simulink model "KVHSerial02"  (R2013a)
settings: Solver=FixedStepDiscrete  StartTime=0.0  StopTime=inf  FixedStep=0.001  RelTol=1e-3
undefined symbols (not defined in the file or in its folder): standard, XOFF, XON
libraries: simulink x2, xpcseriallib x1, xpclib x1, speedgoatlib x1
settings Model: BufferReuse=off  Creator=bgbuss  LastModifiedBy=bgbuss
settings DataIOCC: LimitDataPoints=off  SignalLoggingSaveFormat=ModelDataLogs
settings OptimizationCC: BlockReduction=off  OptimizeBlockIOStorage=off  BufferReuse=off  ExpressionFolding=off  ExpressionDepthLimit=2147483647  LocalBlockOutputs=off
settings DebuggingCC: UnderspecifiedInitializationDetection=Simplified  FcnCallInpInsideContextMsg=EnableAllAsWarning  StrictBusMsg=ErrorOnBusTreatedAsVector
settings HardwareCC: ProdIntDivRoundTo=Zero  ProdEndianess=LittleEndian  ProdHWDeviceType=Generic->32-bit x86 compatible
settings RTWCC: SystemTargetFile=xpctarget.tlc  TemplateMakefile=xpc_default_tmf  Description=xPC Target  ProcessScript=xpctarget_make_rtw_hook
settings xpcTargetCC: TargetFcnLib=ansi_tfl_table_tmw.mat  CodeReplacementLibrary=XPC_BLAS  ParMdlRefBuildCompliant=on  ConcurrentExecutionCompliant=on  CombineSignalStateStructs=off  MATLABClassNameForMDSCustomization=xpcAperiodicCustomization  GRTInterface=on  GenerateAllocFcn=off  RL32LogBufSizeModifier=10000000  xPCTaskExecutionProfile=off  xPCRL32EventNumber=5000  xPCisModelTimeout=off  xPCModelTimeoutSecs=10  xPCLoadParamSetFile=off  xPCConcurrentTasks=off  xPCEnableSFAnimation=off

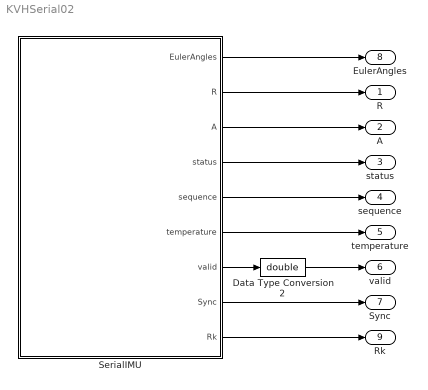
== system KVHSerial02 ==
  Data Type Conversion2 : DataTypeConversion  OutDataTypeStr=double
  SerialIMU : Subsystem
  R : Outport
  A : Outport  Port=2
  status : Outport  Port=3
  sequence : Outport  Port=4
  temperature : Outport  Port=5
  valid : Outport  Port=6
  Sync : Outport  Port=7
  EulerAngles : Outport  Port=8
  Rk : Outport  Port=9
  wires:
  SerialIMU/7(valid) -> Data Type Conversion2/1
  SerialIMU/3(A) -> A/1
  SerialIMU/2(R) -> R/1
  SerialIMU/4(status) -> status/1
  SerialIMU/5(sequence) -> sequence/1
  SerialIMU/6(temperature) -> temperature/1
  SerialIMU/8(Sync) -> Sync/1
  SerialIMU/1(EulerAngles) -> EulerAngles/1
  SerialIMU/9(Rk) -> Rk/1
  Data Type Conversion2/1 -> valid/1

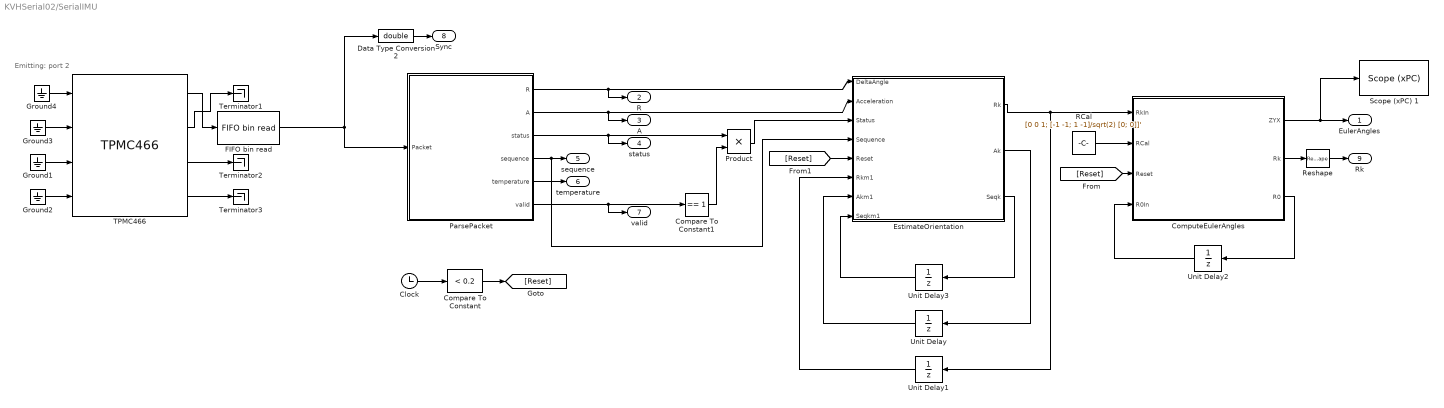
== system KVHSerial02/SerialIMU ==
  note: Emitting: port 2
  Clock : Clock
  Compare To Constant : simulink/Logic and Bit Operations/Compare To Constant  relop=<  const=0.2  OutDataTypeStr=uint8
  Compare To Constant1 : simulink/Logic and Bit Operations/Compare To Constant  relop===  const=1  OutDataTypeStr=uint8
  ComputeEulerAngles : MATLAB Function  TreatAsAtomicUnit=on
  Data Type Conversion2 : DataTypeConversion  OutDataTypeStr=double
  EstimateOrientation : MATLAB Function  TreatAsAtomicUnit=on
  "FIFO bin read " : xpcseriallib/FIFO bin read   header={char([254 129 255 85])}  lengths=[36]  hold=Zero output if no new data  enable=off  maxsize=64  outputtype=8 bit uint null terminated  sampletime=0.001
  Ground{1..4} (4 alike) : Ground
  ParsePacket : Subsystem
  Product : Product  RndMeth=Zero
  RCal : Constant  Value=[0 0 1; [-1 -1; 1 -1]/sqrt(2) [0; 0]]'
  Reshape : Reshape
  Scope (xPC) 1 : xpclib/Misc./Scope (xPC)   scopeno=1  scopetype=Target  autostart=on  viewmode=Graphical rolling  formatstr='%15.6f'  grid=on  ylimits=[-pi pi]  nosamples=500  noprepostsamples=0  interleave=10  triggermode=FreeRun  triggersignal=1  trigsignalfromport=off  triggerlevel=0.0  triggerslope=Either  triggerscope=1  triggersample=0  filename=data.dat  mode=Lazy  writesize=512  autorestart=off  dynamicfilemode=off  maxwritefilesize=512*1024^2
  TPMC466 : speedgoatlib/IO503/TPMC466  group=Basic Setup  port=1  irqnum=9  slot=-1  transceiver1=RS422  standard1=on  baud1=921600  bauddivisor1=1  sampling1=16x (standard)  prescale1=off  parity1=None  ndata1=8  nstop1=1  rlevel1=1  hwmode1=none  swmode1=none  xonchar1=17  xoffchar1=19  rs485auto1=off  rs485delay1=1  xmtfifosize1=1024  xmtdatatype1=8 bit uint null terminated  rcvfifosize1=1024  transceiver2=RS485 half-duplex  standard2=on  baud2=2764800  bauddivisor2=1  sampling2=16x (standard)  prescale2=off  parity2=None  ndata2=8  nstop2=1  rlevel2=quarter full (16)  hwmode2=none  swmode2=XON/XOFF  xonchar2=17  xoffchar2=19  rs485auto2=on  rs485delay2=1  xmtfifosize2=1024  xmtdatatype2=8 bit uint null terminated  rcvfifosize2=1024  transceiver3=RS485 half-duplex  standard3=on  baud3=115200  bauddivisor3=1  sampling3=16x (standard)  prescale3=off  parity3=None  ndata3=8  nstop3=1  rlevel3=half full (32)  hwmode3=none  swmode3=none  xonchar3=17  xoffchar3=19  rs485auto3=off  rs485delay3=0  xmtfifosize3=1024  xmtdatatype3=8 bit uint null terminated  rcvfifosize3=1024  transceiver4=RS485 half-duplex  standard4=on  baud4=115200  bauddivisor4=1  sampling4=16x (standard)  prescale4=off  parity4=None  ndata4=8  nstop4=1  rlevel4=half full (32)  hwmode4=none  swmode4=none  xonchar4=17  xoffchar4=19  rs485auto4=off  rs485delay4=0  xmtfifosize4=1024  xmtdatatype4=8 bit uint null terminated  rcvfifosize4=1024
  Terminator1 : Terminator
  Terminator2 : Terminator
  Terminator3 : Terminator
  Unit Delay : UnitDelay  InitialCondition=[0; 0; 0]  SampleTime=-1
  Unit Delay1 : UnitDelay  InitialCondition=zeros(3,3)  SampleTime=-1
  Unit Delay2 : UnitDelay  InitialCondition=zeros(3,3)  SampleTime=-1
  Unit Delay3 : UnitDelay  SampleTime=-1
  EulerAngles : Outport
  R : Outport  Port=2
  A : Outport  Port=3
  status : Outport  Port=4
  sequence : Outport  Port=5
  temperature : Outport  Port=6
  valid : Outport  Port=7
  Sync : Outport  Port=8
  Rk : Outport  Port=9
  wires:
  ParsePacket/2(A) -> EstimateOrientation/2(Acceleration), A/1
  ParsePacket/1(R) -> EstimateOrientation/1(DeltaAngle), R/1
  ParsePacket/3(status) -> status/1, Product/1
  ParsePacket/4(sequence) -> EstimateOrientation/4(Sequence), sequence/1
  ParsePacket/5(temperature) -> temperature/1
  "FIFO bin read "/1 -> ParsePacket/1(Packet), Data Type Conversion2/1
  ParsePacket/6(valid) -> valid/1, Compare To Constant1/1
  Data Type Conversion2/1 -> Sync/1
  EstimateOrientation/2(Ak) -> Unit Delay/1
  Unit Delay/1 -> EstimateOrientation/7(Akm1)
  EstimateOrientation/1(Rk) -> Unit Delay1/1, ComputeEulerAngles/1(RkIn)
  Unit Delay1/1 -> EstimateOrientation/6(Rkm1)
  [Reset] -> EstimateOrientation/5(Reset)
  RCal/1 -> ComputeEulerAngles/2(RCal)
  Unit Delay2/1 -> ComputeEulerAngles/4(R0In)
  ComputeEulerAngles/1(ZYX) -> Scope (xPC) 1/1, EulerAngles/1
  ComputeEulerAngles/3(R0) -> Unit Delay2/1
  ComputeEulerAngles/2(Rk) -> Reshape/1
  [Reset] -> ComputeEulerAngles/3(Reset)
  Clock/1 -> Compare To Constant/1
  Compare To Constant/1 -> [Reset]
  Reshape/1 -> Rk/1
  Product/1 -> EstimateOrientation/3(Status)
  Compare To Constant1/1 -> Product/2
  Ground4/1 -> TPMC466/1
  Ground3/1 -> TPMC466/2
  Ground1/1 -> TPMC466/3
  Ground2/1 -> TPMC466/4
  TPMC466/3 -> Terminator2/1
  TPMC466/4 -> Terminator3/1
  TPMC466/1 -> "FIFO bin read "/1
  TPMC466/2 -> Terminator1/1
  EstimateOrientation/3(Seqk) -> Unit Delay3/1
  Unit Delay3/1 -> EstimateOrientation/8(Seqkm1)

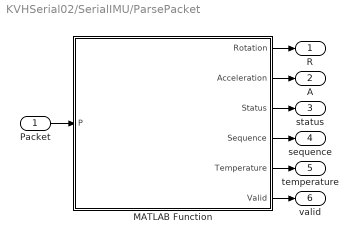
== system KVHSerial02/SerialIMU/ParsePacket ==
  Packet : Inport
  MATLAB Function : MATLAB Function  TreatAsAtomicUnit=on
  R : Outport
  A : Outport  Port=2
  status : Outport  Port=3
  sequence : Outport  Port=4
  temperature : Outport  Port=5
  valid : Outport  Port=6
  wires:
  MATLAB Function/1(Rotation) -> R/1
  MATLAB Function/2(Acceleration) -> A/1
  MATLAB Function/3(Status) -> status/1
  Packet/1 -> MATLAB Function/1(P)
  MATLAB Function/4(Sequence) -> sequence/1
  MATLAB Function/5(Temperature) -> temperature/1
  MATLAB Function/6(Valid) -> valid/1

== matlab function KVHSerial02/SerialIMU/ComputeEulerAngles ==
  data: RkIn input; RCal input; Reset input; R0In input; ZYX output; Rk output; R0 output
function [ZYX, Rk, R0] = fcn(RkIn, RCal, Reset, R0In) %#codegen
    % Convert from IMU frame to robot frame and compute Euler angles. The
    % yaw angle is zeroed whenever (Reset) is true.
        
    if (Reset)
        % Compute the rotation matrix which zeros the initial yaw
        qT0 = M_to_ZYX(RkIn*RCal);
        R0  = Rz(-qT0(1));
    else
        R0 = R0In;
    end
    
    % Transform from IMU to robot frame and zero initial yaw
    Rk = R0*RkIn*RCal;
    
    % Convert Rk to ZYX Euler angles
    ZYX = M_to_ZYX(Rk);
end

function R = Rz(t)
    R = [cos(t) -sin(t) 0; sin(t) cos(t) 0; 0 0 1];
end

== matlab function KVHSerial02/SerialIMU/EstimateOrientation ==
  data: DeltaAngle input; Acceleration input; Status input; Sequence input; Reset input; Rk output; Rkm1 input; Akm1 input; Ak output; Seqkm1 input; Seqk output
function [Rk, Ak, Seqk] = fcn(DeltaAngle,Acceleration,Status,Sequence,Reset,Rkm1,Akm1,Seqkm1) %#codegen
    [Rk, Ak, Seqk] = estimateOrientation(DeltaAngle,Acceleration,Rkm1,Akm1,Status,Sequence,Seqkm1,Reset);
end

== matlab function KVHSerial02/SerialIMU/ParsePacket/MATLAB Function ==
  data: P input; Rotation output; Acceleration output; Status output; Sequence output; Temperature output; Valid output
function [Rotation,Acceleration,Status,Sequence,Temperature,Valid] = KVHParsePacket(P)
    %#codegen
    CMD = [254; 129; 255; 85]; %hex2dec(['FE';'81';'FF';'55']);
    
    Valid = false;
    if all(P(1:4) == CMD)
        Valid = kvhCheckCRC(P(1:36));
    end
    
    Rotation = parseSingle(P(5:16,:));
    Acceleration = parseSingle(P(17:28,:));
    Status = double(P(29));
    Sequence = double(P(30));
    Temperature = parseInt16(P(31:32));
end

function S = parseSingle(D)
    Stmp1 = uint32(reshape(D,4,[]));
    Stmp2 = 16777216*Stmp1(1,:) + 65536*Stmp1(2,:) + 256*Stmp1(3,:) + Stmp1(4,:);
    Stmp3 = typecast(Stmp2,'single');
    S = double(Stmp3');
end

function S = parseInt16(D)
    Stmp1 = uint16(reshape(D,2,[]));
    Stmp2 = 256*Stmp1(1,:) + Stmp1(2,:);
    S = double(Stmp2');
end
